simulink model "homeheater_model"  (R2018a)
settings: Solver=ode45  StartTime=0.0  StopTime=24  RelTol=1e-3
model workspace (MAT data in the model file):
  M_heater_air = 3600
  R_equivalent = 4.329e-07
  T_heater = 50
  T_roomIC = 20
  c_air = 1005.4
  m_room_air = 1470
settings Model: Creator=hirom  LastModifiedBy=hirom
settings OptimizationCC: BlockReduction=off

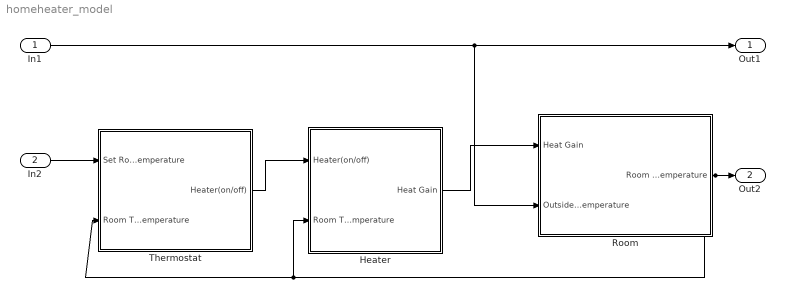
== system homeheater_model ==
  In1 : Inport  Unit=°C
  In2 : Inport  Port=2  Unit=°C
  Heater : Subsystem
  Room : Subsystem
  Thermostat : Subsystem
  Out1 : Outport
  Out2 : Outport  Port=2
  wires:
  Thermostat/1(Heater(on/off)) -> Heater/1(Heater(on/off))
  Heater/1(Heat Gain) -> Room/1(Heat Gain)
  Room/1(Room Temperature) -> Out2/1, Heater/2(Room Temperature), Thermostat/2(Room Temperature)
  In2/1 -> Thermostat/1(Set Room Temperature)
  In1/1 -> Room/2(Outside Temperature), Out1/1

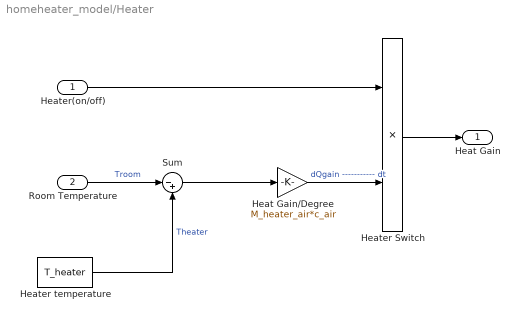
== system homeheater_model/Heater ==
  Heater(on/off) : Inport
  Room Temperature : Inport  Port=2
  Heat Gain/Degree : Gain  Gain=M_heater_air*c_air
  Heater Switch : Product
  Heater temperature : Constant  Value=T_heater
  Sum : Sum  Inputs=|-+
  Heat Gain : Outport  Unit=joule/h
  wires:
  Room Temperature/1 -> Sum/1  "Troom"
  Heater temperature/1 -> Sum/2  "Theater"
  Sum/1 -> Heat Gain/Degree/1
  Heater(on/off)/1 -> Heater Switch/1
  Heat Gain/Degree/1 -> Heater Switch/2  "dQgain ----------- dt"
  Heater Switch/1 -> Heat Gain/1

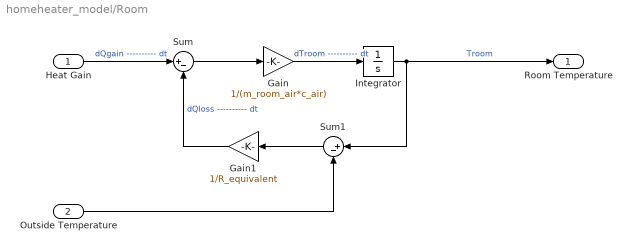
== system homeheater_model/Room ==
  Heat Gain : Inport
  Outside Temperature : Inport  Port=2
  Gain : Gain  Gain=1/(m_room_air*c_air)
  Gain1 : Gain  Gain=1/R_equivalent
  Integrator : Integrator  InitialCondition=T_roomIC
  Sum : Sum  Inputs=|+-
  Sum1 : Sum  Inputs=|+-
  Room Temperature : Outport
  wires:
  Heat Gain/1 -> Sum/1  "dQgain ---------- dt"
  Sum/1 -> Gain/1
  Gain/1 -> Integrator/1  "dTroom ---------- dt"
  Gain1/1 -> Sum/2  "dQloss ---------- dt"
  Integrator/1 -> Sum1/1, Room Temperature/1  "Troom"
  Sum1/1 -> Gain1/1
  Outside Temperature/1 -> Sum1/2

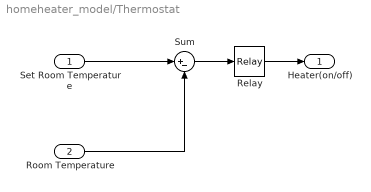
== system homeheater_model/Thermostat ==
  Set Room Temperature : Inport
  Room Temperature : Inport  Port=2
  Relay : Relay  OnSwitchValue=2  OffSwitchValue=-2
  Sum : Sum  Inputs=|+-
  Heater(on/off) : Outport
  wires:
  Set Room Temperature/1 -> Sum/1
  Room Temperature/1 -> Sum/2
  Sum/1 -> Relay/1
  Relay/1 -> Heater(on/off)/1
